simulink model "untitled"  (R2017b)
settings: Solver=VariableStepAuto  StartTime=0.0  StopTime=10.0  RelTol=1e-3
settings Model: Creator=micha  LastModifiedBy=micha

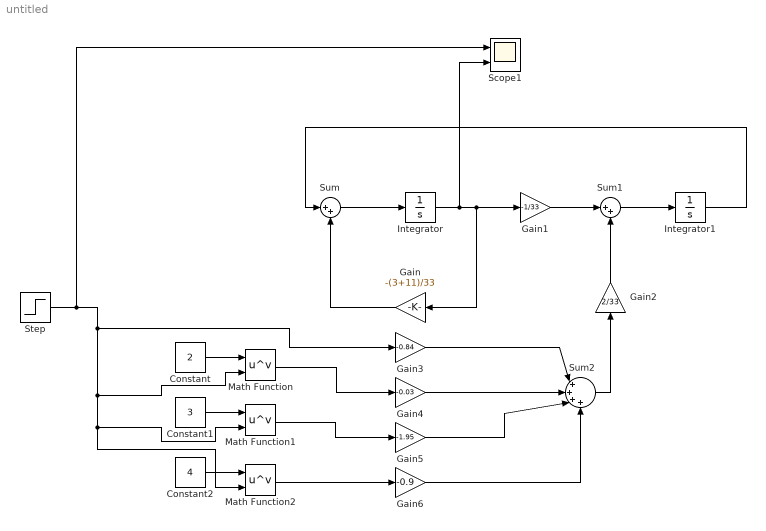
== system untitled ==
  Constant : Constant  Value=2
  Constant1 : Constant  Value=3
  Constant2 : Constant  Value=4
  Gain : Gain  Gain=-(3+11)/33
  Gain1 : Gain  Gain=-1/33
  Gain2 : Gain  Gain=2/33
  Gain3 : Gain  Gain=-0.84
  Gain4 : Gain  Gain=-0.03
  Gain5 : Gain  Gain=-1.95
  Gain6 : Gain  Gain=-0.9
  Integrator : Integrator
  Integrator1 : Integrator
  Math Function : Math  Operator=pow  SaturateOnIntegerOverflow=on
  Math Function1 : Math  Operator=pow  SaturateOnIntegerOverflow=on
  Math Function2 : Math  Operator=pow  SaturateOnIntegerOverflow=on
  Scope1 : Scope  NumInputPorts=2
  Step : Step  SampleTime=0
  Sum : Sum  Inputs=|++
  Sum1 : Sum  Inputs=|++
  Sum2 : Sum  Inputs=|++++
  wires:
  Sum/1 -> Integrator/1
  Gain/1 -> Sum/2
  Integrator/1 -> Scope1/2, Gain/1, Gain1/1
  Gain1/1 -> Sum1/1
  Sum1/1 -> Integrator1/1
  Integrator1/1 -> Sum/1
  Sum2/1 -> Gain2/1
  Gain3/1 -> Sum2/1
  Gain4/1 -> Sum2/2
  Gain6/1 -> Sum2/4
  Gain5/1 -> Sum2/3
  Step/1 -> Scope1/1, Gain3/1, Math Function/2, Math Function1/2, Math Function2/2
  Math Function/1 -> Gain4/1
  Math Function1/1 -> Gain5/1
  Math Function2/1 -> Gain6/1
  Constant/1 -> Math Function/1
  Constant1/1 -> Math Function1/1
  Constant2/1 -> Math Function2/1
  Gain2/1 -> Sum1/2
